simulink model "wlan_phy_tx_pmd"  (Simulink 7.8)
settings: Solver=ode45  StartTime=0.0  StopTime=Sim_Time  RelTol=1e-3
PostLoadFcn:
  | wlan_phy_tx_init
InitFcn:
  | wlan_phy_tx_init
StartFcn:
  | wlan_phy_tx_init
values from neighbouring files (symbols this model uses):
  interleave_64QAM_addr = interleave_64QAM + 2*floor(interleave_64QAM/6)    [wlan_phy_tx_init.m]
  MAX_NUM_BYTES = 4096    [wlan_phy_tx_init.m]
  MAX_NUM_SC = 64    [wlan_phy_tx_init.m]
  Preamble_IQ = PLCP_Preamble.Preamble_t    [wlan_phy_tx_init.m]
  Preamble_IQ_scaled = ALL_MOD_SCALING * Preamble_IQ    [wlan_phy_tx_init.m]
  Sim_Tx_Start_Period = 1*(160 * Tx_Time_usec) + 2e3    [wlan_phy_tx_init.m]
undefined symbols (not defined in the file or in its folder): gcbh, interleave_16QAM, interleave_bpsk, interleave_QPSK, Mod_Constellation_16QAM, Mod_Constellation_64QAM, Mod_Constellation_BPSK, Mod_Constellation_QPSK, xlBlockLoadCallback, xlGetNormalizedPeriod
libraries: xbsIndex_r4 x1173, xbsEDKLib_r4 x1
(part 7 of 8)

== system wlan_phy_tx_pmd/Bit Source/Data Sel 64b/Byte sel ==
  note: Checksum bytes must be output [0,1,2,3], even when they're
      | not aligned to a 32-bit boundary in the actual payload address.
      | This block overrides the payload byte index with a [0,1,2,3]
      | sequence so the CRC bytes are selected in the right order.
  Src Sel : Inport
  Bit Ind : Inport  Port=2
  3LSB : xbsIndex_r4/Slice  nbits=3  boolean_output=off  mode=Lower Bit Location + Width  bit1=0  base1=MSB of Input  bit0=0  base0=LSB of Input  dbl_ovrd=off  block_type=slice
      settings: block_version=8.2.02
  3LSB+3 : xbsIndex_r4/Slice  nbits=3  boolean_output=off  mode=Lower Bit Location + Width  bit1=0  base1=MSB of Input  bit0=3  base0=LSB of Input  dbl_ovrd=off  block_type=slice
      settings: block_version=8.2.02
  Constant1 : xbsIndex_r4/Constant  const=0  gui_display_data_type=Fixed-point  arith_type=Unsigned  n_bits=2  bin_pt=0  preci_type=Single  exp_width=8  frac_width=24  explicit_period=off  period=1  equ=P=C  opselect=C  inp2=PCIN>>17  opr=+  inp1=P  carry=CIN  dbl_ovrd=off  block_type=constant
      settings: block_version=VER_STRING_GOES_HERE
  Constant2 : xbsIndex_r4/Constant  const=7  gui_display_data_type=Fixed-point  arith_type=Unsigned  n_bits=3  bin_pt=0  preci_type=Single  exp_width=8  frac_width=24  explicit_period=off  period=1  equ=P=C  opselect=C  inp2=PCIN>>17  opr=+  inp1=P  carry=CIN  dbl_ovrd=off  block_type=constant
      settings: block_version=VER_STRING_GOES_HERE
  Counter : xbsIndex_r4/Counter  cnt_type=Free Running  cnt_to=Inf  operation=Up  start_count=0  cnt_by_val=1  arith_type=Unsigned  n_bits=2  bin_pt=0  load_pin=off  rst=on  en=on  explicit_period=off  period=1  dbl_ovrd=off  use_behavioral_HDL=off  implementation=Fabric  block_type=counter
  Delay : xbsIndex_r4/Delay  rst=off  infoeditControl=Selection of Reset will increase slice count due to use of real FFs and instead of SRLs  en=off  latency=1  dbl_ovrd=off  reg_retiming=off  block_type=delay
  LSB : xbsIndex_r4/Slice  nbits=1  boolean_output=on  mode=Lower Bit Location + Width  bit1=0  base1=MSB of Input  bit0=0  base0=LSB of Input  dbl_ovrd=off  block_type=slice
      settings: block_version=8.2.02
  Logical1 : xbsIndex_r4/Logical  logical_function=AND  inputs=3  en=off  latency=0  precision=Full  arith_type=Unsigned  n_bits=16  bin_pt=0  align_bp=on  dbl_ovrd=off  block_type=logical
  Mux : xbsIndex_r4/Mux  inputs=3  en=off  latency=0  precision=Full  arith_type=Unsigned  n_bits=16  bin_pt=14  quantization=Truncate  overflow=Wrap  dbl_ovrd=off  block_type=mux
  Posedge : Subsystem
  Relational3 : xbsIndex_r4/Relational  mode=a=b  en=off  latency=0  dbl_ovrd=off  block_type=relational
  Sel : Outport
  wires:
  Delay/1 -> Logical1/3
  LSB/1 -> Logical1/1
  Logical1/1 -> Posedge/1(D)
  Posedge/1(Q) -> Counter/2
  [TX_RESET] -> Counter/1
  Mux/1 -> Sel/1
  Constant1/1 -> Mux/4
  Counter/1 -> Mux/3
  Relational3/1 -> Delay/1, Logical1/2
  Constant2/1 -> Relational3/2
  3LSB/1 -> Relational3/1
  Src Sel/1 -> LSB/1, Mux/1
  3LSB+3/1 -> Mux/2
  Bit Ind/1 -> 3LSB/1, 3LSB+3/1

== system wlan_phy_tx_pmd/Bit Source/Data Sel 64b/CRC Byte En ==
  note: SERVICE is not included
      | in CRC calculation
  DATA : Inport
  Bit Valid : Inport  Port=2
  bit sel : Inport  Port=3
  Constant3 : xbsIndex_r4/Constant  const=0  gui_display_data_type=Fixed-point  arith_type=Unsigned  n_bits=2  bin_pt=0  preci_type=Single  exp_width=8  frac_width=24  explicit_period=off  period=1  equ=P=C  opselect=C  inp2=PCIN>>17  opr=+  inp1=P  carry=CIN  dbl_ovrd=off  block_type=constant
      settings: block_version=VER_STRING_GOES_HERE
  Logical : xbsIndex_r4/Logical  logical_function=AND  inputs=2  en=off  latency=0  precision=Full  arith_type=Unsigned  n_bits=16  bin_pt=0  align_bp=on  dbl_ovrd=off  block_type=logical
  Logical1 : xbsIndex_r4/Logical  logical_function=AND  inputs=2  en=off  latency=0  precision=Full  arith_type=Unsigned  n_bits=16  bin_pt=0  align_bp=on  dbl_ovrd=off  block_type=logical
  Relational1 : xbsIndex_r4/Relational  mode=a=b  en=off  latency=0  dbl_ovrd=off  block_type=relational
  Skip First 2 : Subsystem
  Byte En : Outport
  wires:
  Skip First 2/1(" En[2+]") -> Byte En/1
  Logical1/1 -> Skip First 2/1(En)
  bit sel/1 -> Relational1/2
  Logical/1 -> Logical1/1
  Constant3/1 -> Relational1/1
  Relational1/1 -> Logical1/2
  Bit Valid/1 -> Logical/2
  DATA/1 -> Logical/1

== system wlan_phy_tx_pmd/Bit Source/Data Sel 64b/CRC32 Calc ==
  byte_valid : Inport
  byte : Inport  Port=2
  24LSB : xbsIndex_r4/Slice  nbits=24  boolean_output=off  mode=Lower Bit Location + Width  bit1=0  base1=MSB of Input  bit0=0  base0=LSB of Input  dbl_ovrd=off  block_type=slice
      settings: infoedit="Extracts a given range of bits from each input sample and presents it at the output.  The output type is ordinarily unsigned with binary point at zero, but can be Boolean when the slice is one bit wide.<P><P>Hardware notes: In hardware this block costs nothing."  block_version=VER_STRING_GOES_HERE
  8MSB : xbsIndex_r4/Slice  nbits=8  boolean_output=off  mode=Upper Bit Location + Width  bit1=0  base1=MSB of Input  bit0=0  base0=LSB of Input  dbl_ovrd=off  block_type=slice
      settings: infoedit="Extracts a given range of bits from each input sample and presents it at the output.  The output type is ordinarily unsigned with binary point at zero, but can be Boolean when the slice is one bit wide.<P><P>Hardware notes: In hardware this block costs nothing."  block_version=VER_STRING_GOES_HERE
  Assert1 : xbsIndex_r4/Assert  assert_type=off  type_source=Explicitly  gui_display_data_type=Fixed-point  arith_type="Signed  (2's comp)"  n_bits=16  bin_pt=14  preci_type=Single  exp_width=8  frac_width=24  assert_rate=on  rate_source=Explicitly  period=1  output_port=on  block_type=assert
      settings: block_version=VER_STRING_GOES_HERE
  B0 : xbsIndex_r4/Slice  nbits=8  boolean_output=off  mode=Lower Bit Location + Width  bit1=0  base1=MSB of Input  bit0=0  base0=LSB of Input  dbl_ovrd=off  block_type=slice
  B1 : xbsIndex_r4/Slice  nbits=8  boolean_output=off  mode=Lower Bit Location + Width  bit1=0  base1=MSB of Input  bit0=8  base0=LSB of Input  dbl_ovrd=off  block_type=slice
  B2 : xbsIndex_r4/Slice  nbits=8  boolean_output=off  mode=Lower Bit Location + Width  bit1=0  base1=MSB of Input  bit0=16  base0=LSB of Input  dbl_ovrd=off  block_type=slice
  B3 : xbsIndex_r4/Slice  nbits=8  boolean_output=off  mode=Lower Bit Location + Width  bit1=0  base1=MSB of Input  bit0=24  base0=LSB of Input  dbl_ovrd=off  block_type=slice
  CRC Calc : Scope  NumInputPorts=7
      settings: TimeRange=10000  YMin=0~0~0~0~0~0~-0.1  YMax=250~1~1~1~25~1~1.1  SaveName=ScopeData17
  CRC Remainders1 : xbsIndex_r4/ROM  depth=256  initVector=CRC_Table32  distributed_mem=Distributed memory  rst=off  init_reg=0  en=off  latency=0  gui_display_data_type=Fixed-point  arith_type=Unsigned  n_bits=32  bin_pt=0  preci_type=Single  exp_width=8  frac_width=24  dbl_ovrd=off  optimize=Area  use_rpm=off  block_type=sprom
      settings: xl_area=[0, 0, 0, 0, 0, 0, 0]  block_version=VER_STRING_GOES_HERE
  Concat : xbsIndex_r4/Concat  num_inputs=4  dbl_ovrd=off  block_type=concat
  Concat1 : xbsIndex_r4/Concat  num_inputs=2  dbl_ovrd=off  block_type=concat
      settings: block_version=VER_STRING_GOES_HERE
  Constant1 : xbsIndex_r4/Constant  const=0  gui_display_data_type=Fixed-point  arith_type=Unsigned  n_bits=8  bin_pt=0  preci_type=Single  exp_width=8  frac_width=24  explicit_period=off  period=1  equ=P=C  opselect=C  inp2=PCIN>>17  opr=+  inp1=P  carry=CIN  dbl_ovrd=off  block_type=constant
      settings: block_version=VER_STRING_GOES_HERE
  Endian Swap : Subsystem
  Endian Swap1 : Subsystem
  Endian Swap2 : Subsystem
  Endian Swap3 : Subsystem
  Endian Swap4 : Subsystem
  Gateway Out3 : xbsIndex_r4/Gateway Out  inherit_from_input=off  hdl_port=off  timing_constraint=None  locs_specified=off  LOCs={}  UseAsDAC=off  DACChannel='1'  block_type=gatewayout
  Gateway Out4 : xbsIndex_r4/Gateway Out  inherit_from_input=off  hdl_port=off  timing_constraint=None  locs_specified=off  LOCs={}  UseAsDAC=off  DACChannel='1'  block_type=gatewayout
  Inverter : xbsIndex_r4/Inverter  en=off  latency=0  dbl_ovrd=off  block_type=inv
  Logical3 : xbsIndex_r4/Logical  logical_function=XOR  inputs=2  en=off  latency=0  precision=Full  arith_type=Unsigned  n_bits=8  bin_pt=2  align_bp=on  dbl_ovrd=off  block_type=logical
      settings: xl_area=[0, 0, 0, 0, 0, 0, 0]  block_version=VER_STRING_GOES_HERE
  Logical4 : xbsIndex_r4/Logical  logical_function=XOR  inputs=2  en=off  latency=0  precision=Full  arith_type=Unsigned  n_bits=8  bin_pt=2  align_bp=on  dbl_ovrd=off  block_type=logical
      settings: xl_area=[0, 0, 0, 0, 0, 0, 0]  block_version=VER_STRING_GOES_HERE
  crc_accum : xbsIndex_r4/Register  init=hex2dec('FFFFFFFF')  rst=on  en=on  dbl_ovrd=off  block_type=register
      settings: xl_area=[0, 0, 0, 0, 0, 0, 0]  block_version=VER_STRING_GOES_HERE
  CRC32 : Outport
  wires:
  Inverter/1 -> B0/1, B1/1, B3/1, B2/1
  Endian Swap4/1(I) -> Concat/4
  Endian Swap3/1(I) -> Concat/3
  Endian Swap2/1(I) -> Concat/2
  Endian Swap1/1(I) -> Concat/1
  Endian Swap/1(I) -> Logical3/2
  Gateway Out4/1 -> CRC Calc/1  "Byte"
  Gateway Out3/1 -> CRC Calc/2  "Byte Valid"
  Concat/1 -> CRC32/1
  B3/1 -> Endian Swap4/1(B)
  B2/1 -> Endian Swap3/1(B)
  B1/1 -> Endian Swap2/1(B)
  B0/1 -> Endian Swap1/1(B)
  byte/1 -> Endian Swap/1(B), Gateway Out4/1
  8MSB/1 -> Logical3/1
  24LSB/1 -> Concat1/1
  [TX_RESET] -> crc_accum/2
  byte_valid/1 -> Gateway Out3/1, crc_accum/3
  Assert1/1 -> Inverter/1, 8MSB/1, 24LSB/1
  crc_accum/1 -> Assert1/1
  Logical4/1 -> crc_accum/1
  Constant1/1 -> Concat1/2
  Concat1/1 -> Logical4/1
  CRC Remainders1/1 -> Logical4/2
  Logical3/1 -> CRC Remainders1/1

== system wlan_phy_tx_pmd/Bit Source/Data Sel 64b/Timestamp Insert ==
  Data : Inport
  Bit Ind : Inport  Port=2
  Concat1 : xbsIndex_r4/Concat  num_inputs=2  dbl_ovrd=off  block_type=concat
  Constant : Constant  Value=hex2dec('04030201')
  Constant1 : Constant  Value=hex2dec('08070605')
  Gateway Out{1..4} (4 alike) : xbsIndex_r4/Gateway Out  inherit_from_input=off  hdl_port=off  timing_constraint=None  locs_specified=off  LOCs={}  UseAsDAC=off  DACChannel='1'  block_type=gatewayout
  Logical1 : xbsIndex_r4/Logical  logical_function=AND  inputs=2  en=off  latency=0  precision=Full  arith_type=Unsigned  n_bits=16  bin_pt=0  align_bp=on  dbl_ovrd=off  block_type=logical
  MAC_Timestamp_LSB : xbsIndex_r4/Gateway In  gui_display_data_type=Fixed-point  arith_type=Unsigned  n_bits=32  bin_pt=0  preci_type=Single  exp_width=8  frac_width=24  quantization="Round  (unbiased: +/- Inf)"  overflow=Saturate  period=1  dbl_ovrd=off  timing_constraint=None  locs_specified=off  LOCs={}  UseAsADC=off  ADCChannel='1'  inherit_from_input=off  hdl_port=on  block_type=gatewayin
      settings: block_version=VER_STRING_GOES_HERE
  MAC_Timestamp_MSB : xbsIndex_r4/Gateway In  gui_display_data_type=Fixed-point  arith_type=Unsigned  n_bits=32  bin_pt=0  preci_type=Single  exp_width=8  frac_width=24  quantization="Round  (unbiased: +/- Inf)"  overflow=Saturate  period=1  dbl_ovrd=off  timing_constraint=None  locs_specified=off  LOCs={}  UseAsADC=off  ADCChannel='1'  inherit_from_input=off  hdl_port=on  block_type=gatewayin
      settings: block_version=VER_STRING_GOES_HERE
  MSB : xbsIndex_r4/Slice  nbits=ceil(log2(MAX_NUM_BYTES))  boolean_output=off  mode=Upper Bit Location + Width  bit1=0  base1=MSB of Input  bit0=0  base0=LSB of Input  dbl_ovrd=off  block_type=slice
      settings: block_version=8.2.02
  Mux1 : xbsIndex_r4/Mux  inputs=2  en=off  latency=0  precision=Full  arith_type=Unsigned  n_bits=16  bin_pt=14  quantization=Truncate  overflow=Wrap  dbl_ovrd=off  block_type=mux
  Relational1 : xbsIndex_r4/Relational  mode=a<=b  en=off  latency=0  dbl_ovrd=off  block_type=relational
  Relational3 : xbsIndex_r4/Relational  mode=a>=b  en=off  latency=0  dbl_ovrd=off  block_type=relational
  Timestamp insert : Scope  NumInputPorts=7
      settings: TimeRange=10000  YMin=0~0~0~0~-0.1~0~-0.1  YMax=1~1~1~1~1.1~1~1.1  SaveName=ScopeData26
  reg1 : xbsIndex_r4/Register  init=0  rst=off  en=off  dbl_ovrd=off  block_type=register
      settings: xl_area=[0, 0, 0, 0, 0, 0, 0]  block_version=VER_STRING_GOES_HERE
  reg2 : xbsIndex_r4/Register  init=0  rst=off  en=off  dbl_ovrd=off  block_type=register
      settings: xl_area=[0, 0, 0, 0, 0, 0, 0]  block_version=VER_STRING_GOES_HERE
  Tx Data : Outport
  wires:
  MAC_Timestamp_MSB/1 -> reg1/1
  MAC_Timestamp_LSB/1 -> reg2/1
  reg1/1 -> Concat1/1
  reg2/1 -> Concat1/2
  Concat1/1 -> Mux1/3
  Bit Ind/1 -> MSB/1, Gateway Out1/1
  Data/1 -> Mux1/2
  Mux1/1 -> Tx Data/1, Gateway Out3/1
  MSB/1 -> Relational3/1, Relational1/1, Gateway Out4/1  "Byte Index"
  [regTx_Timestamp_Ins_StartByte] -> Relational3/2
  [regTx_Timestamp_Ins_EndByte] -> Relational1/2
  Relational3/1 -> Logical1/1
  Relational1/1 -> Logical1/2
  Logical1/1 -> Mux1/1, Gateway Out2/1
  Constant/1 -> MAC_Timestamp_LSB/1
  Constant1/1 -> MAC_Timestamp_MSB/1
  Gateway Out4/1 -> Timestamp insert/2  "Byte Addr"
  Gateway Out1/1 -> Timestamp insert/1  "Bit Addr"
  Gateway Out2/1 -> Timestamp insert/3  "Mux Sel"
  Gateway Out3/1 -> Timestamp insert/4  "Tx Data"

== system wlan_phy_tx_pmd/Bit Source/SIGNAL Capture/Posedge ==
  D : Inport
  Delay : xbsIndex_r4/Delay  rst=off  infoeditControl=Selection of Reset will increase slice count due to use of real FFs and instead of SRLs  en=off  latency=1  dbl_ovrd=off  reg_retiming=off  block_type=delay
      settings: infoedit=Hardware notes: A delay line is a chain, each link of which is an SRL16 followed by a flip-flop. If register retiming is enabled, the delay line is a chain of flip-flops.  xl_area=[1 1 0 0 0 0 0]  block_version=VER_STRING_GOES_HERE
  Inverter : xbsIndex_r4/Inverter  en=off  latency=0  dbl_ovrd=off  block_type=inv
      settings: xl_area=[0 0 0 0 0 0 0]  block_version=VER_STRING_GOES_HERE
  Logical1 : xbsIndex_r4/Logical  logical_function=AND  inputs=2  en=off  latency=0  precision=Full  arith_type=Unsigned  n_bits=8  bin_pt=2  align_bp=on  dbl_ovrd=off  block_type=logical
      settings: xl_area=[1 0 0 1 0 0 0]  block_version=VER_STRING_GOES_HERE
  Q : Outport
  wires:
  D/1 -> Logical1/2, Delay/1
  Logical1/1 -> Q/1
  Inverter/1 -> Logical1/1
  Delay/1 -> Inverter/1

== system wlan_phy_tx_pmd/Bit Source/SIGNAL Capture/SIGNAL Slice ==
  note: 6-bit TAIL - always 0
  S : Inport
  Concat : xbsIndex_r4/Concat  num_inputs=2  dbl_ovrd=off  block_type=concat
  Constant : xbsIndex_r4/Constant  const=0  gui_display_data_type=Fixed-point  arith_type=Unsigned  n_bits=10  bin_pt=0  preci_type=Single  exp_width=8  frac_width=24  explicit_period=off  period=1  equ=P=C  opselect=C  inp2=PCIN>>17  opr=+  inp1=P  carry=CIN  dbl_ovrd=off  block_type=constant
  Constant1 : xbsIndex_r4/Constant  const=0  gui_display_data_type=Fixed-point  arith_type=Unsigned  n_bits=2  bin_pt=0  preci_type=Single  exp_width=8  frac_width=24  explicit_period=off  period=1  equ=P=C  opselect=C  inp2=PCIN>>17  opr=+  inp1=P  carry=CIN  dbl_ovrd=off  block_type=constant
  Endian Swap4 : Subsystem
  Gateway Out{1..3,6} (4 alike) : xbsIndex_r4/Gateway Out  inherit_from_input=off  hdl_port=off  timing_constraint=None  locs_specified=off  LOCs={}  UseAsDAC=off  DACChannel='1'  block_type=gatewayout
  Logical5 : xbsIndex_r4/Logical  logical_function=OR  inputs=2  en=off  latency=0  precision=Full  arith_type=Unsigned  n_bits=16  bin_pt=0  align_bp=on  dbl_ovrd=off  block_type=logical
  Relational1 : xbsIndex_r4/Relational  mode=a!=b  en=off  latency=0  dbl_ovrd=off  block_type=relational
  Relational2 : xbsIndex_r4/Relational  mode=a>b  en=off  latency=0  dbl_ovrd=off  block_type=relational
  SIGNAL Decode : Scope  NumInputPorts=4
      settings: YMin=0~5~87.5~-5  YMax=140000~9~130~5  SaveName=ScopeData24
  b[16:5] : xbsIndex_r4/Slice  nbits=12  boolean_output=off  mode=Lower Bit Location + Width  bit1=0  base1=MSB of Input  bit0=5  base0=LSB of Input  dbl_ovrd=off  block_type=slice
  b[23:18] : xbsIndex_r4/Slice  nbits=6  boolean_output=off  mode=Lower Bit Location + Width  bit1=0  base1=MSB of Input  bit0=18  base0=LSB of Input  dbl_ovrd=off  block_type=slice
  b[3:0] : xbsIndex_r4/Slice  nbits=4  boolean_output=off  mode=Lower Bit Location + Width  bit1=0  base1=MSB of Input  bit0=0  base0=LSB of Input  dbl_ovrd=off  block_type=slice
  LENGTH : Outport
  RATE : Outport  Port=2
  invalid : Outport  Port=3
  wires:
  S/1 -> b[3:0]/1, b[16:5]/1, b[23:18]/1, Gateway Out6/1
  b[3:0]/1 -> Endian Swap4/1(B)
  b[16:5]/1 -> Relational2/1, LENGTH/1, Gateway Out2/1
  b[23:18]/1 -> Relational1/1
  Concat/1 -> Relational2/2
  Relational2/1 -> Logical5/1
  Constant1/1 -> Relational1/2
  Relational1/1 -> Logical5/2
  Logical5/1 -> invalid/1, Gateway Out3/1
  Endian Swap4/1(I) -> RATE/1, Gateway Out1/1
  Gateway Out6/1 -> SIGNAL Decode/1
  Gateway Out1/1 -> SIGNAL Decode/2
  Gateway Out2/1 -> SIGNAL Decode/3
  Gateway Out3/1 -> SIGNAL Decode/4
  [regTx_SIGNAL_MAX_LENGTH_KB] -> Concat/1
  Constant/1 -> Concat/2

== system wlan_phy_tx_pmd/Bit Source/Sym Compute Ctrl/Posedge ==
  D : Inport
  Delay : xbsIndex_r4/Delay  rst=off  infoeditControl=Selection of Reset will increase slice count due to use of real FFs and instead of SRLs  en=off  latency=1  dbl_ovrd=off  reg_retiming=off  block_type=delay
      settings: infoedit=Hardware notes: A delay line is a chain, each link of which is an SRL16 followed by a flip-flop. If register retiming is enabled, the delay line is a chain of flip-flops.  xl_area=[1 1 0 0 0 0 0]  block_version=VER_STRING_GOES_HERE
  Inverter : xbsIndex_r4/Inverter  en=off  latency=0  dbl_ovrd=off  block_type=inv
      settings: xl_area=[0 0 0 0 0 0 0]  block_version=VER_STRING_GOES_HERE
  Logical1 : xbsIndex_r4/Logical  logical_function=AND  inputs=2  en=off  latency=0  precision=Full  arith_type=Unsigned  n_bits=8  bin_pt=2  align_bp=on  dbl_ovrd=off  block_type=logical
      settings: xl_area=[1 0 0 1 0 0 0]  block_version=VER_STRING_GOES_HERE
  Q : Outport
  wires:
  D/1 -> Logical1/2, Delay/1
  Logical1/1 -> Q/1
  Inverter/1 -> Logical1/1
  Delay/1 -> Inverter/1

== system wlan_phy_tx_pmd/Bit Source/Sym Compute Ctrl/Posedge1 ==
  D : Inport
  Delay : xbsIndex_r4/Delay  rst=off  infoeditControl=Selection of Reset will increase slice count due to use of real FFs and instead of SRLs  en=off  latency=1  dbl_ovrd=off  reg_retiming=off  block_type=delay
      settings: infoedit=Hardware notes: A delay line is a chain, each link of which is an SRL16 followed by a flip-flop. If register retiming is enabled, the delay line is a chain of flip-flops.  xl_area=[1 1 0 0 0 0 0]  block_version=VER_STRING_GOES_HERE
  Inverter : xbsIndex_r4/Inverter  en=off  latency=0  dbl_ovrd=off  block_type=inv
      settings: xl_area=[0 0 0 0 0 0 0]  block_version=VER_STRING_GOES_HERE
  Logical1 : xbsIndex_r4/Logical  logical_function=AND  inputs=2  en=off  latency=0  precision=Full  arith_type=Unsigned  n_bits=8  bin_pt=2  align_bp=on  dbl_ovrd=off  block_type=logical
      settings: xl_area=[1 0 0 1 0 0 0]  block_version=VER_STRING_GOES_HERE
  Q : Outport
  wires:
  Delay/1 -> Inverter/1
  Logical1/1 -> Q/1
  D/1 -> Delay/1, Logical1/2
  Inverter/1 -> Logical1/1

== system wlan_phy_tx_pmd/Bit Source/Sym Compute Ctrl/Posedge2 ==
  D : Inport
  Delay : xbsIndex_r4/Delay  rst=off  infoeditControl=Selection of Reset will increase slice count due to use of real FFs and instead of SRLs  en=off  latency=1  dbl_ovrd=off  reg_retiming=off  block_type=delay
      settings: infoedit=Hardware notes: A delay line is a chain, each link of which is an SRL16 followed by a flip-flop. If register retiming is enabled, the delay line is a chain of flip-flops.  xl_area=[1 1 0 0 0 0 0]  block_version=VER_STRING_GOES_HERE
  Inverter : xbsIndex_r4/Inverter  en=off  latency=0  dbl_ovrd=off  block_type=inv
      settings: xl_area=[0 0 0 0 0 0 0]  block_version=VER_STRING_GOES_HERE
  Logical1 : xbsIndex_r4/Logical  logical_function=AND  inputs=2  en=off  latency=0  precision=Full  arith_type=Unsigned  n_bits=8  bin_pt=2  align_bp=on  dbl_ovrd=off  block_type=logical
      settings: xl_area=[1 0 0 1 0 0 0]  block_version=VER_STRING_GOES_HERE
  Q : Outport
  wires:
  Inverter/1 -> Logical1/1
  D/1 -> Logical1/2, Delay/1
  Logical1/1 -> Q/1
  Delay/1 -> Inverter/1

== system wlan_phy_tx_pmd/Bit Source/Sym Compute Ctrl/S-R Latch ==
  S : Inport
  R : Inport  Port=2
  Constant1 : xbsIndex_r4/Constant  const=1  gui_display_data_type=Fixed-point  arith_type=Boolean  n_bits=1  bin_pt=0  preci_type=Single  exp_width=8  frac_width=24  explicit_period=off  period=1  equ=P=C  opselect=C  inp2=PCIN>>17  opr=+  inp1=P  carry=CIN  dbl_ovrd=off  block_type=constant
      settings: block_version=VER_STRING_GOES_HERE
  Convert1 : xbsIndex_r4/Convert  gui_display_data_type=Boolean  arith_type=Boolean  n_bits=1  bin_pt=0  float_type=Single  exp_bits=8  fraction_bits=24  quantization=Truncate  overflow=Wrap  en=off  latency=0  dbl_ovrd=off  pipeline=off  block_type=convert
  Convert2 : xbsIndex_r4/Convert  gui_display_data_type=Boolean  arith_type=Boolean  n_bits=1  bin_pt=0  float_type=Single  exp_bits=8  fraction_bits=24  quantization=Truncate  overflow=Wrap  en=off  latency=0  dbl_ovrd=off  pipeline=off  block_type=convert
  Register2 : xbsIndex_r4/Register  init=0  rst=on  en=on  dbl_ovrd=off  block_type=register
      settings: xl_area=[1 1 0 0 0 0 0]  block_version=VER_STRING_GOES_HERE
  Q : Outport
  wires:
  Convert2/1 -> Register2/3
  Convert1/1 -> Register2/2
  Constant1/1 -> Register2/1
  R/1 -> Convert1/1
  Register2/1 -> Q/1
  S/1 -> Convert2/1

== system wlan_phy_tx_pmd/Bit Source/Sym Compute Ctrl/S-R Latch1 ==
  S : Inport
  R : Inport  Port=2
  Constant1 : xbsIndex_r4/Constant  const=1  gui_display_data_type=Fixed-point  arith_type=Boolean  n_bits=1  bin_pt=0  preci_type=Single  exp_width=8  frac_width=24  explicit_period=off  period=1  equ=P=C  opselect=C  inp2=PCIN>>17  opr=+  inp1=P  carry=CIN  dbl_ovrd=off  block_type=constant
      settings: block_version=VER_STRING_GOES_HERE
  Convert1 : xbsIndex_r4/Convert  gui_display_data_type=Boolean  arith_type=Boolean  n_bits=1  bin_pt=0  float_type=Single  exp_bits=8  fraction_bits=24  quantization=Truncate  overflow=Wrap  en=off  latency=0  dbl_ovrd=off  pipeline=off  block_type=convert
  Convert2 : xbsIndex_r4/Convert  gui_display_data_type=Boolean  arith_type=Boolean  n_bits=1  bin_pt=0  float_type=Single  exp_bits=8  fraction_bits=24  quantization=Truncate  overflow=Wrap  en=off  latency=0  dbl_ovrd=off  pipeline=off  block_type=convert
  Register2 : xbsIndex_r4/Register  init=0  rst=on  en=on  dbl_ovrd=off  block_type=register
      settings: xl_area=[1 1 0 0 0 0 0]  block_version=VER_STRING_GOES_HERE
  Q : Outport
  wires:
  S/1 -> Convert2/1
  Register2/1 -> Q/1
  R/1 -> Convert1/1
  Constant1/1 -> Register2/1
  Convert1/1 -> Register2/2
  Convert2/1 -> Register2/3

== system wlan_phy_tx_pmd/Interleave & Modulate/16-QAM/16QAM Int Addr ==
  New Sym : Inport
  Bit Valid : Inport  Port=2
  16QAM Ind : xbsIndex_r4/ROM  depth=length(interleave_16QAM)  initVector=interleave_16QAM  distributed_mem=Block RAM  rst=off  init_reg=0  en=off  latency=1  gui_display_data_type=Fixed-point  arith_type=Unsigned  n_bits=8  bin_pt=0  preci_type=Single  exp_width=8  frac_width=24  dbl_ovrd=off  optimize=Area  use_rpm=on  block_type=sprom
  Constant2 : xbsIndex_r4/Constant  const=191  gui_display_data_type=Fixed-point  arith_type=Unsigned  n_bits=8  bin_pt=0  preci_type=Single  exp_width=8  frac_width=24  explicit_period=off  period=1  equ=P=C  opselect=C  inp2=PCIN>>17  opr=+  inp1=P  carry=CIN  dbl_ovrd=off  block_type=constant
  Counter : xbsIndex_r4/Counter  cnt_type=Count Limited  cnt_to=191  operation=Up  start_count=0  cnt_by_val=1  arith_type=Unsigned  n_bits=8  bin_pt=0  load_pin=off  rst=on  en=on  explicit_period=off  period=4  dbl_ovrd=off  use_behavioral_HDL=off  implementation=Fabric  block_type=counter
  Delay2 : xbsIndex_r4/Delay  rst=off  infoeditControl=Selection of Reset will increase slice count due to use of real FFs and instead of SRLs  en=off  latency=1  dbl_ovrd=off  reg_retiming=off  block_type=delay
  Logical1 : xbsIndex_r4/Logical  logical_function=OR  inputs=3  en=off  latency=0  precision=Full  arith_type=Unsigned  n_bits=16  bin_pt=0  align_bp=on  dbl_ovrd=off  block_type=logical
  Logical2 : xbsIndex_r4/Logical  logical_function=AND  inputs=2  en=off  latency=0  precision=Full  arith_type=Unsigned  n_bits=16  bin_pt=0  align_bp=on  dbl_ovrd=off  block_type=logical
  Osc : Subsystem
  Posedge : Subsystem
  Relational2 : xbsIndex_r4/Relational  mode=a=b  en=off  latency=0  dbl_ovrd=off  block_type=relational
  Wr Offset : Outport
  Wr Addr : Outport  Port=2
  wires:
  16QAM Ind/1 -> Wr Addr/1
  Constant2/1 -> Relational2/2
  Counter/1 -> Relational2/1, 16QAM Ind/1
  Posedge/1(Q) -> Osc/2(En), Logical1/3
  Logical1/1 -> Counter/1
  New Sym/1 -> Logical1/2
  Osc/1(Q) -> Delay2/1
  Bit Valid/1 -> Counter/2, Logical2/1
  [TX_RESET] -> Osc/1(R), Logical1/1
  Delay2/1 -> Wr Offset/1
  Logical2/1 -> Posedge/1(D)
  Relational2/1 -> Logical2/2

== system wlan_phy_tx_pmd/Interleave & Modulate/64-QAM/64QAM Int Addr ==
  New Sym : Inport
  Bit Valid : Inport  Port=2
  64QAM Ind : xbsIndex_r4/ROM  depth=length(interleave_64QAM_addr)  initVector=interleave_64QAM_addr  distributed_mem=Block RAM  rst=off  init_reg=0  en=off  latency=1  gui_display_data_type=Fixed-point  arith_type=Unsigned  n_bits=9  bin_pt=0  preci_type=Single  exp_width=8  frac_width=24  dbl_ovrd=off  optimize=Area  use_rpm=on  block_type=sprom
  Constant2 : xbsIndex_r4/Constant  const=287  gui_display_data_type=Fixed-point  arith_type=Unsigned  n_bits=9  bin_pt=0  preci_type=Single  exp_width=8  frac_width=24  explicit_period=off  period=1  equ=P=C  opselect=C  inp2=PCIN>>17  opr=+  inp1=P  carry=CIN  dbl_ovrd=off  block_type=constant
  Counter : xbsIndex_r4/Counter  cnt_type=Count Limited  cnt_to=287  operation=Up  start_count=0  cnt_by_val=1  arith_type=Unsigned  n_bits=9  bin_pt=0  load_pin=off  rst=on  en=on  explicit_period=off  period=4  dbl_ovrd=off  use_behavioral_HDL=off  implementation=Fabric  block_type=counter
  Delay2 : xbsIndex_r4/Delay  rst=off  infoeditControl=Selection of Reset will increase slice count due to use of real FFs and instead of SRLs  en=off  latency=1  dbl_ovrd=off  reg_retiming=off  block_type=delay
  Logical1 : xbsIndex_r4/Logical  logical_function=OR  inputs=3  en=off  latency=0  precision=Full  arith_type=Unsigned  n_bits=16  bin_pt=0  align_bp=on  dbl_ovrd=off  block_type=logical
  Logical2 : xbsIndex_r4/Logical  logical_function=AND  inputs=2  en=off  latency=0  precision=Full  arith_type=Unsigned  n_bits=16  bin_pt=0  align_bp=on  dbl_ovrd=off  block_type=logical
  Osc : Subsystem
  Posedge : Subsystem
  Relational2 : xbsIndex_r4/Relational  mode=a=b  en=off  latency=0  dbl_ovrd=off  block_type=relational
  Wr Offset : Outport
  Wr Addr : Outport  Port=2
  wires:
  Relational2/1 -> Logical2/2
  Logical2/1 -> Posedge/1(D)
  Delay2/1 -> Wr Offset/1
  [TX_RESET] -> Logical1/1, Osc/1(R)
  Bit Valid/1 -> Logical2/1, Counter/2
  Osc/1(Q) -> Delay2/1
  New Sym/1 -> Logical1/2
  Logical1/1 -> Counter/1
  Posedge/1(Q) -> Logical1/3, Osc/2(En)
  Counter/1 -> 64QAM Ind/1, Relational2/1
  Constant2/1 -> Relational2/2
  64QAM Ind/1 -> Wr Addr/1

== system wlan_phy_tx_pmd/Interleave & Modulate/BPSK/BPSK Int Addr ==
  New Sym : Inport
  Bit Valid : Inport  Port=2
  BPSK Int : xbsIndex_r4/ROM  depth=length(interleave_bpsk)  initVector=interleave_bpsk  distributed_mem=Block RAM  rst=off  init_reg=0  en=off  latency=1  gui_display_data_type=Fixed-point  arith_type=Unsigned  n_bits=6  bin_pt=0  preci_type=Single  exp_width=8  frac_width=24  dbl_ovrd=off  optimize=Area  use_rpm=on  block_type=sprom
  Constant2 : xbsIndex_r4/Constant  const=47  gui_display_data_type=Fixed-point  arith_type=Unsigned  n_bits=6  bin_pt=0  preci_type=Single  exp_width=8  frac_width=24  explicit_period=off  period=1  equ=P=C  opselect=C  inp2=PCIN>>17  opr=+  inp1=P  carry=CIN  dbl_ovrd=off  block_type=constant
  Counter : xbsIndex_r4/Counter  cnt_type=Count Limited  cnt_to=47  operation=Up  start_count=0  cnt_by_val=1  arith_type=Unsigned  n_bits=6  bin_pt=0  load_pin=off  rst=on  en=on  explicit_period=off  period=4  dbl_ovrd=off  use_behavioral_HDL=off  implementation=Fabric  block_type=counter
  Delay2 : xbsIndex_r4/Delay  rst=off  infoeditControl=Selection of Reset will increase slice count due to use of real FFs and instead of SRLs  en=off  latency=1  dbl_ovrd=off  reg_retiming=off  block_type=delay
  Logical1 : xbsIndex_r4/Logical  logical_function=OR  inputs=3  en=off  latency=0  precision=Full  arith_type=Unsigned  n_bits=16  bin_pt=0  align_bp=on  dbl_ovrd=off  block_type=logical
  Logical2 : xbsIndex_r4/Logical  logical_function=AND  inputs=2  en=off  latency=0  precision=Full  arith_type=Unsigned  n_bits=16  bin_pt=0  align_bp=on  dbl_ovrd=off  block_type=logical
  Osc : Subsystem
  Posedge : Subsystem
  Relational2 : xbsIndex_r4/Relational  mode=a=b  en=off  latency=0  dbl_ovrd=off  block_type=relational
  Wr Offset : Outport
  Wr Addr : Outport  Port=2
  wires:
  Constant2/1 -> Relational2/2
  Counter/1 -> Relational2/1, BPSK Int/1
  Posedge/1(Q) -> Osc/2(En), Logical1/3
  Logical1/1 -> Counter/1
  New Sym/1 -> Logical1/2
  Osc/1(Q) -> Delay2/1
  Bit Valid/1 -> Counter/2, Logical2/1
  [TX_RESET] -> Osc/1(R), Logical1/1
  BPSK Int/1 -> Wr Addr/1
  Delay2/1 -> Wr Offset/1
  Logical2/1 -> Posedge/1(D)
  Relational2/1 -> Logical2/2

== system wlan_phy_tx_pmd/Interleave & Modulate/Coded Bit Counter/S-R Latch2 ==
  S : Inport
  R : Inport  Port=2
  Constant1 : xbsIndex_r4/Constant  const=1  gui_display_data_type=Fixed-point  arith_type=Boolean  n_bits=1  bin_pt=0  preci_type=Single  exp_width=8  frac_width=24  explicit_period=off  period=1  equ=P=C  opselect=C  inp2=PCIN>>17  opr=+  inp1=P  carry=CIN  dbl_ovrd=off  block_type=constant
      settings: block_version=VER_STRING_GOES_HERE
  Convert1 : xbsIndex_r4/Convert  gui_display_data_type=Boolean  arith_type=Boolean  n_bits=1  bin_pt=0  float_type=Single  exp_bits=8  fraction_bits=24  quantization=Truncate  overflow=Wrap  en=off  latency=0  dbl_ovrd=off  pipeline=off  block_type=convert
  Convert2 : xbsIndex_r4/Convert  gui_display_data_type=Boolean  arith_type=Boolean  n_bits=1  bin_pt=0  float_type=Single  exp_bits=8  fraction_bits=24  quantization=Truncate  overflow=Wrap  en=off  latency=0  dbl_ovrd=off  pipeline=off  block_type=convert
  Register2 : xbsIndex_r4/Register  init=0  rst=on  en=on  dbl_ovrd=off  block_type=register
      settings: xl_area=[1 1 0 0 0 0 0]  block_version=VER_STRING_GOES_HERE
  Q : Outport
  wires:
  Convert2/1 -> Register2/3
  Convert1/1 -> Register2/2
  Constant1/1 -> Register2/1
  R/1 -> Convert1/1
  Register2/1 -> Q/1
  S/1 -> Convert2/1

== system wlan_phy_tx_pmd/Interleave & Modulate/Control & Pilots/Data SC Map ==
  sc_ind : Inport
  Constant2 : xbsIndex_r4/Constant  const=MAX_NUM_SC  gui_display_data_type=Fixed-point  arith_type=Unsigned  n_bits=ceil(log2(MAX_NUM_SC))+1  bin_pt=0  preci_type=Single  exp_width=8  frac_width=24  explicit_period=off  period=1  equ=P=C  opselect=C  inp2=PCIN>>17  opr=+  inp1=P  carry=CIN  dbl_ovrd=off  block_type=constant
  Relational1 : xbsIndex_r4/Relational  mode=a!=b  en=off  latency=0  dbl_ovrd=off  block_type=relational
  SC Sym Map : xbsIndex_r4/ROM  depth=MAX_NUM_SC  initVector=sc_data_sym_map  distributed_mem=Distributed memory  rst=off  init_reg=0  en=off  latency=0  gui_display_data_type=Fixed-point  arith_type=Unsigned  n_bits=ceil(log2(MAX_NUM_SC))+1  bin_pt=0  preci_type=Single  exp_width=8  frac_width=24  dbl_ovrd=off  optimize=Area  use_rpm=on  block_type=sprom
  Slice : xbsIndex_r4/Slice  nbits=ceil(log2(MAX_NUM_SC))  boolean_output=off  mode=Lower Bit Location + Width  bit1=0  base1=MSB of Input  bit0=0  base0=LSB of Input  dbl_ovrd=off  block_type=slice
  data_sym_ind : Outport
  data_sym_valid : Outport  Port=2
  wires:
  sc_ind/1 -> SC Sym Map/1
  Constant2/1 -> Relational1/1
  SC Sym Map/1 -> Relational1/2, Slice/1
  Relational1/1 -> data_sym_valid/1
  Slice/1 -> data_sym_ind/1

== system wlan_phy_tx_pmd/Interleave & Modulate/Control & Pilots/Pilot Gen ==
  sc_ind : Inport
  reset : Inport  Port=2
  Constant1 : xbsIndex_r4/Constant  const=Mod_Constellation_BPSK(1)  gui_display_data_type=Fixed-point  arith_type=Signed (2's comp)  n_bits=12  bin_pt=11  preci_type=Single  exp_width=8  frac_width=24  explicit_period=off  period=1  equ=P=C  opselect=C  inp2=PCIN>>17  opr=+  inp1=P  carry=CIN  dbl_ovrd=off  block_type=constant
  Constant5 : xbsIndex_r4/Constant  const=Mod_Constellation_BPSK(2)  gui_display_data_type=Fixed-point  arith_type=Signed (2's comp)  n_bits=12  bin_pt=11  preci_type=Single  exp_width=8  frac_width=24  explicit_period=off  period=1  equ=P=C  opselect=C  inp2=PCIN>>17  opr=+  inp1=P  carry=CIN  dbl_ovrd=off  block_type=constant
  Delay : xbsIndex_r4/Delay  rst=off  infoeditControl=Selection of Reset will increase slice count due to use of real FFs and instead of SRLs  en=off  latency=1  dbl_ovrd=off  reg_retiming=off  block_type=delay
  Logical : xbsIndex_r4/Logical  logical_function=XOR  inputs=2  en=off  latency=0  precision=Full  arith_type=Unsigned  n_bits=8  bin_pt=2  align_bp=on  dbl_ovrd=off  block_type=logical
      settings: xl_area=[0, 0, 0, 0, 0, 0, 0]  block_version=VER_STRING_GOES_HERE
  Mux1 : xbsIndex_r4/Mux  inputs=2  en=off  latency=0  precision=Full  arith_type="Signed  (2's comp)"  n_bits=8  bin_pt=2  quantization=Truncate  overflow=Wrap  dbl_ovrd=off  block_type=mux
      settings: xl_area=[16 0 0 32 0 0 0]  block_version=VER_STRING_GOES_HERE
  Pilot Selection : Subsystem
  Posedge : Subsystem
  Relational1 : xbsIndex_r4/Relational  mode=a<b  en=off  latency=0  dbl_ovrd=off  block_type=relational
  Scrambling LFSR : Subsystem
  pilot_valid : Outport
  Pilot_I : Outport  Port=2
  wires:
  Pilot Selection/1(Pilot) -> pilot_valid/1
  Pilot Selection/2(Negate) -> Logical/1
  sc_ind/1 -> Pilot Selection/1(sc_ind), Delay/1, Relational1/1
  Delay/1 -> Relational1/2
  Relational1/1 -> Posedge/1(D)
  Posedge/1(Q) -> Scrambling LFSR/1(en)
  Scrambling LFSR/1(Q) -> Logical/2
  Logical/1 -> Mux1/1
  Constant5/1 -> Mux1/2
  Constant1/1 -> Mux1/3
  Mux1/1 -> Pilot_I/1
  reset/1 -> Scrambling LFSR/2(rst)

== system wlan_phy_tx_pmd/Interleave & Modulate/Control & Pilots/Posedge ==
  note: Rising Edge Detection
  D : Inport
  Delay : xbsIndex_r4/Delay  rst=off  infoeditControl=Selection of Reset will increase slice count due to use of real FFs and instead of SRLs  en=off  latency=1  dbl_ovrd=off  reg_retiming=off  block_type=delay
      settings: infoedit=Hardware notes: A delay line is a chain, each link of which is an SRL16 followed by a flip-flop. If register retiming is enabled, the delay line is a chain of flip-flops.  xl_area=[1 1 0 0 0 0 0]  block_version=VER_STRING_GOES_HERE
  Inverter : xbsIndex_r4/Inverter  en=off  latency=0  dbl_ovrd=off  block_type=inv
      settings: xl_area=[0 0 0 0 0 0 0]  block_version=VER_STRING_GOES_HERE
  Logical1 : xbsIndex_r4/Logical  logical_function=AND  inputs=2  en=off  latency=0  precision=Full  arith_type=Unsigned  n_bits=8  bin_pt=2  align_bp=on  dbl_ovrd=off  block_type=logical
      settings: xl_area=[1 0 0 1 0 0 0]  block_version=VER_STRING_GOES_HERE
  Q : Outport
  wires:
  D/1 -> Logical1/2, Delay/1
  Logical1/1 -> Q/1
  Inverter/1 -> Logical1/1
  Delay/1 -> Inverter/1

== system wlan_phy_tx_pmd/Interleave & Modulate/Control & Pilots/Posedge1 ==
  note: Rising Edge Detection
  D : Inport
  Delay : xbsIndex_r4/Delay  rst=off  infoeditControl=Selection of Reset will increase slice count due to use of real FFs and instead of SRLs  en=off  latency=1  dbl_ovrd=off  reg_retiming=off  block_type=delay
      settings: infoedit=Hardware notes: A delay line is a chain, each link of which is an SRL16 followed by a flip-flop. If register retiming is enabled, the delay line is a chain of flip-flops.  xl_area=[1 1 0 0 0 0 0]  block_version=VER_STRING_GOES_HERE
  Inverter : xbsIndex_r4/Inverter  en=off  latency=0  dbl_ovrd=off  block_type=inv
      settings: xl_area=[0 0 0 0 0 0 0]  block_version=VER_STRING_GOES_HERE
  Logical1 : xbsIndex_r4/Logical  logical_function=AND  inputs=2  en=off  latency=0  precision=Full  arith_type=Unsigned  n_bits=8  bin_pt=2  align_bp=on  dbl_ovrd=off  block_type=logical
      settings: xl_area=[1 0 0 1 0 0 0]  block_version=VER_STRING_GOES_HERE
  Q : Outport
  wires:
  Delay/1 -> Inverter/1
  Inverter/1 -> Logical1/1
  Logical1/1 -> Q/1
  D/1 -> Delay/1, Logical1/2

== system wlan_phy_tx_pmd/Interleave & Modulate/Control & Pilots/S-R Latch1 ==
  S : Inport
  R : Inport  Port=2
  Constant1 : xbsIndex_r4/Constant  const=1  gui_display_data_type=Fixed-point  arith_type=Boolean  n_bits=1  bin_pt=0  preci_type=Single  exp_width=8  frac_width=24  explicit_period=off  period=1  equ=P=C  opselect=C  inp2=PCIN>>17  opr=+  inp1=P  carry=CIN  dbl_ovrd=off  block_type=constant
      settings: block_version=VER_STRING_GOES_HERE
  Convert1 : xbsIndex_r4/Convert  gui_display_data_type=Boolean  arith_type=Boolean  n_bits=1  bin_pt=0  float_type=Single  exp_bits=8  fraction_bits=24  quantization=Truncate  overflow=Wrap  en=off  latency=0  dbl_ovrd=off  pipeline=off  block_type=convert
  Convert2 : xbsIndex_r4/Convert  gui_display_data_type=Boolean  arith_type=Boolean  n_bits=1  bin_pt=0  float_type=Single  exp_bits=8  fraction_bits=24  quantization=Truncate  overflow=Wrap  en=off  latency=0  dbl_ovrd=off  pipeline=off  block_type=convert
  Register2 : xbsIndex_r4/Register  init=0  rst=on  en=on  dbl_ovrd=off  block_type=register
      settings: xl_area=[1 1 0 0 0 0 0]  block_version=VER_STRING_GOES_HERE
  Q : Outport
  wires:
  Convert2/1 -> Register2/3
  Convert1/1 -> Register2/2
  Constant1/1 -> Register2/1
  R/1 -> Convert1/1
  Register2/1 -> Q/1
  S/1 -> Convert2/1

== system wlan_phy_tx_pmd/Interleave & Modulate/Control & Pilots/S-R Latch2 ==
  S : Inport
  R : Inport  Port=2
  Constant1 : xbsIndex_r4/Constant  const=1  gui_display_data_type=Boolean  arith_type=Boolean  n_bits=1  bin_pt=0  preci_type=Single  exp_width=8  frac_width=24  explicit_period=off  period=1  equ=P=C  opselect=C  inp2=PCIN>>17  opr=+  inp1=P  carry=CIN  dbl_ovrd=off  block_type=constant
      settings: block_version=VER_STRING_GOES_HERE
  Convert1 : xbsIndex_r4/Convert  gui_display_data_type=Boolean  arith_type=Boolean  n_bits=1  bin_pt=0  float_type=Single  exp_bits=8  fraction_bits=24  quantization=Truncate  overflow=Wrap  en=off  latency=0  dbl_ovrd=off  pipeline=off  block_type=convert
  Convert2 : xbsIndex_r4/Convert  gui_display_data_type=Boolean  arith_type=Boolean  n_bits=1  bin_pt=0  float_type=Single  exp_bits=8  fraction_bits=24  quantization=Truncate  overflow=Wrap  en=off  latency=0  dbl_ovrd=off  pipeline=off  block_type=convert
  Register2 : xbsIndex_r4/Register  init=0  rst=on  en=on  dbl_ovrd=off  block_type=register
      settings: xl_area=[1 1 0 0 0 0 0]  block_version=VER_STRING_GOES_HERE
  Q : Outport
  wires:
  Convert2/1 -> Register2/3
  Convert1/1 -> Register2/2
  Constant1/1 -> Register2/1
  R/1 -> Convert1/1
  Register2/1 -> Q/1
  S/1 -> Convert2/1

== system wlan_phy_tx_pmd/Interleave & Modulate/Control & Pilots/Subcarrier Index Count ==
  en : Inport
  reset : Inport  Port=2
  AddSub : xbsIndex_r4/AddSub  mode=Subtraction  use_carryin=off  use_carryout=off  en=off  latency=0  precision=Full  arith_type=Unsigned  n_bits=16  bin_pt=14  quantization=Truncate  overflow=Wrap  dbl_ovrd=off  use_behavioral_HDL=off  hw_selection=Fabric  pipelined=off  block_type=addsub
  Constant1 : xbsIndex_r4/Constant  const=1  gui_display_data_type=Fixed-point  arith_type=Unsigned  n_bits=1  bin_pt=0  preci_type=Single  exp_width=8  frac_width=24  explicit_period=off  period=1  equ=P=C  opselect=C  inp2=PCIN>>17  opr=+  inp1=P  carry=CIN  dbl_ovrd=off  block_type=constant
  Logical1 : xbsIndex_r4/Logical  logical_function=AND  inputs=2  en=off  latency=0  precision=Full  arith_type=Unsigned  n_bits=16  bin_pt=0  align_bp=on  dbl_ovrd=off  block_type=logical
  Logical2 : xbsIndex_r4/Logical  logical_function=OR  inputs=2  en=off  latency=0  precision=Full  arith_type=Unsigned  n_bits=16  bin_pt=0  align_bp=on  dbl_ovrd=off  block_type=logical
  Relational3 : xbsIndex_r4/Relational  mode=a=b  en=off  latency=0  dbl_ovrd=off  block_type=relational
  Subcarrier Index : xbsIndex_r4/Counter  cnt_type=Free Running  cnt_to=47  operation=Up  start_count=0  cnt_by_val=1  arith_type=Unsigned  n_bits=ceil(log2(MAX_NUM_SC))  bin_pt=0  load_pin=off  rst=on  en=on  explicit_period=off  period=4  dbl_ovrd=off  use_behavioral_HDL=off  implementation=Fabric  block_type=counter
  sc_ind : Outport
  last : Outport  Port=2
  wires:
  Subcarrier Index/1 -> Relational3/2, sc_ind/1
  AddSub/1 -> Relational3/1
  Relational3/1 -> Logical1/1
  en/1 -> Subcarrier Index/2, Logical1/2
  Logical2/1 -> Subcarrier Index/1
  reset/1 -> Logical2/1
  Logical1/1 -> Logical2/2, last/1
  [regTx_NUM_SC] -> AddSub/1
  Constant1/1 -> AddSub/2

== system wlan_phy_tx_pmd/Interleave & Modulate/QPSK/QPSK Int Addr ==
  New Sym : Inport
  Bit Valid : Inport  Port=2
  Constant2 : xbsIndex_r4/Constant  const=95  gui_display_data_type=Fixed-point  arith_type=Unsigned  n_bits=7  bin_pt=0  preci_type=Single  exp_width=8  frac_width=24  explicit_period=off  period=1  equ=P=C  opselect=C  inp2=PCIN>>17  opr=+  inp1=P  carry=CIN  dbl_ovrd=off  block_type=constant
  Counter : xbsIndex_r4/Counter  cnt_type=Count Limited  cnt_to=95  operation=Up  start_count=0  cnt_by_val=1  arith_type=Unsigned  n_bits=7  bin_pt=0  load_pin=off  rst=on  en=on  explicit_period=off  period=4  dbl_ovrd=off  use_behavioral_HDL=off  implementation=Fabric  block_type=counter
  Delay2 : xbsIndex_r4/Delay  rst=off  infoeditControl=Selection of Reset will increase slice count due to use of real FFs and instead of SRLs  en=off  latency=1  dbl_ovrd=off  reg_retiming=off  block_type=delay
  Logical1 : xbsIndex_r4/Logical  logical_function=OR  inputs=3  en=off  latency=0  precision=Full  arith_type=Unsigned  n_bits=16  bin_pt=0  align_bp=on  dbl_ovrd=off  block_type=logical
  Logical2 : xbsIndex_r4/Logical  logical_function=AND  inputs=2  en=off  latency=0  precision=Full  arith_type=Unsigned  n_bits=16  bin_pt=0  align_bp=on  dbl_ovrd=off  block_type=logical
  Osc : Subsystem
  Posedge : Subsystem
  QPSK Int1 : xbsIndex_r4/ROM  depth=length(interleave_QPSK)  initVector=interleave_QPSK  distributed_mem=Block RAM  rst=off  init_reg=0  en=off  latency=1  gui_display_data_type=Fixed-point  arith_type=Unsigned  n_bits=7  bin_pt=0  preci_type=Single  exp_width=8  frac_width=24  dbl_ovrd=off  optimize=Area  use_rpm=on  block_type=sprom
  Relational2 : xbsIndex_r4/Relational  mode=a=b  en=off  latency=0  dbl_ovrd=off  block_type=relational
  Wr Offset : Outport
  Wr Addr : Outport  Port=2
  wires:
  QPSK Int1/1 -> Wr Addr/1
  Constant2/1 -> Relational2/2
  Counter/1 -> Relational2/1, QPSK Int1/1
  Posedge/1(Q) -> Osc/2(En), Logical1/3
  Logical1/1 -> Counter/1
  New Sym/1 -> Logical1/2
  Osc/1(Q) -> Delay2/1
  Bit Valid/1 -> Counter/2, Logical2/1
  [TX_RESET] -> Osc/1(R), Logical1/1
  Delay2/1 -> Wr Offset/1
  Logical2/1 -> Posedge/1(D)
  Relational2/1 -> Logical2/2

== system wlan_phy_tx_pmd/Preamble & Outputs/DAC Outputs/Ant Enables ==
  Logical{1,3,5,7} (4 alike) : xbsIndex_r4/Logical  logical_function=AND  inputs=2  en=off  latency=0  precision=Full  arith_type=Unsigned  n_bits=16  bin_pt=0  align_bp=on  dbl_ovrd=off  block_type=logical
  Logical{2,4,6,8} (4 alike) : xbsIndex_r4/Logical  logical_function=OR  inputs=2  en=off  latency=0  precision=Full  arith_type=Unsigned  n_bits=16  bin_pt=0  align_bp=on  dbl_ovrd=off  block_type=logical
  b0 : xbsIndex_r4/Slice  nbits=1  boolean_output=on  mode=Lower Bit Location + Width  bit1=0  base1=MSB of Input  bit0=0  base0=LSB of Input  dbl_ovrd=off  block_type=slice
  b1 : xbsIndex_r4/Slice  nbits=1  boolean_output=on  mode=Lower Bit Location + Width  bit1=0  base1=MSB of Input  bit0=1  base0=LSB of Input  dbl_ovrd=off  block_type=slice
  b2 : xbsIndex_r4/Slice  nbits=1  boolean_output=on  mode=Lower Bit Location + Width  bit1=0  base1=MSB of Input  bit0=2  base0=LSB of Input  dbl_ovrd=off  block_type=slice
  b3 : xbsIndex_r4/Slice  nbits=1  boolean_output=on  mode=Lower Bit Location + Width  bit1=0  base1=MSB of Input  bit0=3  base0=LSB of Input  dbl_ovrd=off  block_type=slice
  A En : Outport
  B En : Outport  Port=2
  C En : Outport  Port=3
  D En : Outport  Port=4
  wires:
  [regTx_AntA_Tx_En] -> Logical2/1
  Logical2/1 -> A En/1
  [MAC_Tx_Ant_Mask] -> b0/1, b1/1, b2/1, b3/1
  Logical1/1 -> Logical2/2
  [regTx_Use_MAC_Ant_Masks] -> Logical1/2, Logical3/2, Logical5/2, Logical7/2
  b0/1 -> Logical1/1
  Logical3/1 -> Logical4/2
  [regTx_AntB_Tx_En] -> Logical4/1
  b1/1 -> Logical3/1
  Logical5/1 -> Logical6/2
  [regTx_AntC_Tx_En] -> Logical6/1
  b2/1 -> Logical5/1
  Logical7/1 -> Logical8/2
  [regTx_AntD_Tx_En] -> Logical8/1
  Logical4/1 -> B En/1
  Logical6/1 -> C En/1
  b3/1 -> Logical7/1
  Logical8/1 -> D En/1

== system wlan_phy_tx_pmd/Preamble & Outputs/FIFO/I/Q Concat ==
  I : Inport
  Q : Inport  Port=2
  Concat : xbsIndex_r4/Concat  num_inputs=2  dbl_ovrd=off  block_type=concat
  Convert : xbsIndex_r4/Convert  gui_display_data_type=Fixed-point  arith_type="Signed  (2's comp)"  n_bits=16  bin_pt=15  float_type=Single  exp_bits=8  fraction_bits=24  quantization=Truncate  overflow=Saturate  en=off  latency=0  dbl_ovrd=off  pipeline=off  block_type=convert
  Convert1 : xbsIndex_r4/Convert  gui_display_data_type=Fixed-point  arith_type="Signed  (2's comp)"  n_bits=16  bin_pt=15  float_type=Single  exp_bits=8  fraction_bits=24  quantization=Truncate  overflow=Saturate  en=off  latency=0  dbl_ovrd=off  pipeline=off  block_type=convert
  FFT Clip : Scope  NumInputPorts=4
      settings: TimeRange=30000  YMin=0~0~0~-0.1  YMax=300~300~1~1.1  SaveName=ScopeData11
  Gateway Out{1..3,14} (4 alike) : xbsIndex_r4/Gateway Out  inherit_from_input=off  hdl_port=off  timing_constraint=None  locs_specified=off  LOCs={}  UseAsDAC=off  DACChannel='1'  block_type=gatewayout
  Reinterpret : xbsIndex_r4/Reinterpret  force_arith_type=on  arith_type=Unsigned  force_bin_pt=on  bin_pt=0  block_type=reinterpret
  Reinterpret1 : xbsIndex_r4/Reinterpret  force_arith_type=on  arith_type=Unsigned  force_bin_pt=on  bin_pt=0  block_type=reinterpret
  IQ : Outport
  wires:
  Q/1 -> Convert1/1, Gateway Out1/1
  Concat/1 -> IQ/1
  I/1 -> Convert/1, Gateway Out14/1
  Reinterpret1/1 -> Concat/2
  Reinterpret/1 -> Concat/1
  Convert/1 -> Reinterpret/1, Gateway Out3/1
  Convert1/1 -> Reinterpret1/1, Gateway Out2/1
  Gateway Out14/1 -> FFT Clip/1
  Gateway Out1/1 -> FFT Clip/2
  Gateway Out3/1 -> FFT Clip/3
  Gateway Out2/1 -> FFT Clip/4

== system wlan_phy_tx_pmd/Preamble & Outputs/FIFO/I/Q Slice ==
  IQ : Inport
  Reinterpret2 : xbsIndex_r4/Reinterpret  force_arith_type=on  arith_type="Signed  (2's comp)"  force_bin_pt=on  bin_pt=15  block_type=reinterpret
  Reinterpret3 : xbsIndex_r4/Reinterpret  force_arith_type=on  arith_type="Signed  (2's comp)"  force_bin_pt=on  bin_pt=15  block_type=reinterpret
  Slice : xbsIndex_r4/Slice  nbits=16  boolean_output=off  mode=Upper Bit Location + Width  bit1=0  base1=MSB of Input  bit0=0  base0=LSB of Input  dbl_ovrd=off  block_type=slice
  Slice1 : xbsIndex_r4/Slice  nbits=16  boolean_output=off  mode=Lower Bit Location + Width  bit1=0  base1=MSB of Input  bit0=0  base0=LSB of Input  dbl_ovrd=off  block_type=slice
  I : Outport
  Q : Outport  Port=2
  wires:
  Slice/1 -> Reinterpret2/1
  Slice1/1 -> Reinterpret3/1
  IQ/1 -> Slice1/1, Slice/1
  Reinterpret2/1 -> I/1
  Reinterpret3/1 -> Q/1
